simulink model "PID_Linear_gain"  (R2022a)
settings: Solver=VariableStepAuto  StartTime=0.0  StopTime=10.0  RelTol=1e-3
settings Model: Creator=Reza  LastModifiedBy=Reza

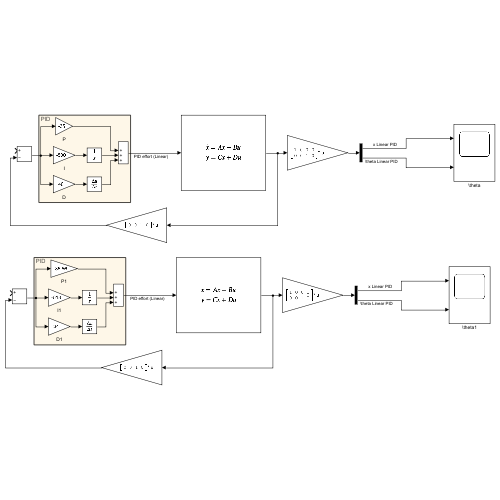
[thumbnail: Simulink's stored preview of the top-level diagram]
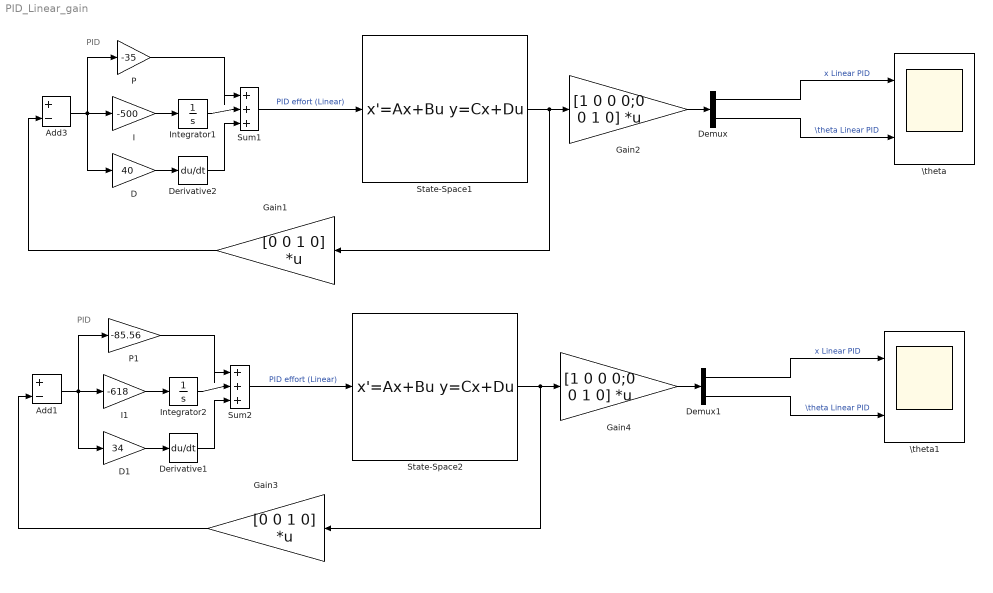
== system PID_Linear_gain ==
  note: PID
  note: PID
  Add1 : Sum  Inputs=+-
  Add3 : Sum  Inputs=+-
  D : Gain  Gain=40
  D1 : Gain  Gain=34
  Demux : Demux  Outputs=2
  Demux1 : Demux  Outputs=2
  Derivative1 : Derivative
  Derivative2 : Derivative
  Gain1 : Gain  Gain=[0 0 1 0]  Multiplication=Matrix(K*u)
  Gain2 : Gain  Gain=[1 0 0 0;0 0 1 0]  Multiplication=Matrix(K*u)
  Gain3 : Gain  Gain=[0 0 1 0]  Multiplication=Matrix(K*u)
  Gain4 : Gain  Gain=[1 0 0 0;0 0 1 0]  Multiplication=Matrix(K*u)
  I : Gain  Gain=-500
  I1 : Gain  Gain=-618
  Integrator1 : Integrator
  Integrator2 : Integrator
  P : Gain  Gain=-35
  P1 : Gain  Gain=-85.56
  State-Space1 : StateSpace  A="[0 1 0 0;163.2653   88.1633  405.0653  121.1633;0 0 0 1;-163.2653  -88.1633 -395.2653 -121.1633]"  B=[0;0.5;0;-0.5]  C=eye(4)  D=[0;0;0;0]  InitialCondition=[0;0;10*pi/180;0]
  State-Space2 : StateSpace  A="[0 1 0 0;163.2653   88.1633  405.0653  121.1633;0 0 0 1;-163.2653  -88.1633 -395.2653 -121.1633]"  B=[0;0.5;0;-0.5]  C=eye(4)  D=[0;0;0;0]  InitialCondition=[0;0;10*pi/180;0]
  Sum1 : Sum  Inputs=|+++
  Sum2 : Sum  Inputs=|+++
  \theta : Scope  NumInputPorts=2
  \theta1 : Scope  NumInputPorts=2
  wires:
  Demux/1 -> \theta/1  "x Linear PID"
  Gain2/1 -> Demux/1
  Demux/2 -> \theta/2  "\\theta Linear PID"
  State-Space1/1 -> Gain1/1, Gain2/1
  Gain1/1 -> Add3/2
  D/1 -> Derivative2/1
  Integrator1/1 -> Sum1/2
  Add3/1 -> D/1, I/1, P/1
  Derivative2/1 -> Sum1/3
  I/1 -> Integrator1/1
  P/1 -> Sum1/1
  Sum1/1 -> State-Space1/1  "PID effort (Linear)"
  Sum2/1 -> State-Space2/1  "PID effort (Linear)"
  P1/1 -> Sum2/1
  I1/1 -> Integrator2/1
  Derivative1/1 -> Sum2/3
  Add1/1 -> P1/1, I1/1, D1/1
  Integrator2/1 -> Sum2/2
  D1/1 -> Derivative1/1
  Gain3/1 -> Add1/2
  State-Space2/1 -> Gain4/1, Gain3/1
  Demux1/2 -> \theta1/2  "\\theta Linear PID"
  Gain4/1 -> Demux1/1
  Demux1/1 -> \theta1/1  "x Linear PID"
